simulink model "system2"  (R2023b)
settings: Solver=FixedStepAuto  StartTime=0.0  StopTime=Tmdl  FixedStep=Tmdl/n_steps  RelTol=1e-3
undefined symbols (not defined in the file): x1_initial, x2_initial, x3_initial
settings Model: Creator=deniskirbaba  LastModifiedBy=deniskirbaba

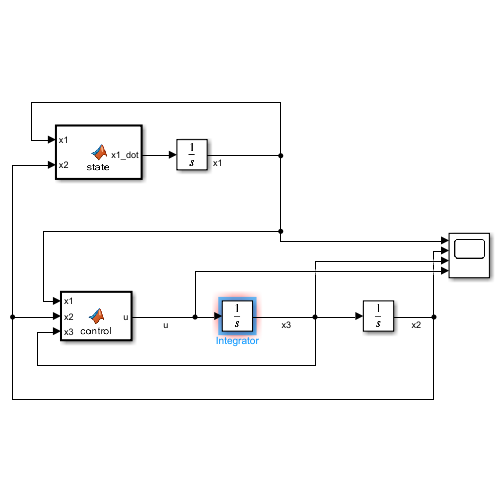
[thumbnail: Simulink's stored preview of the top-level diagram]
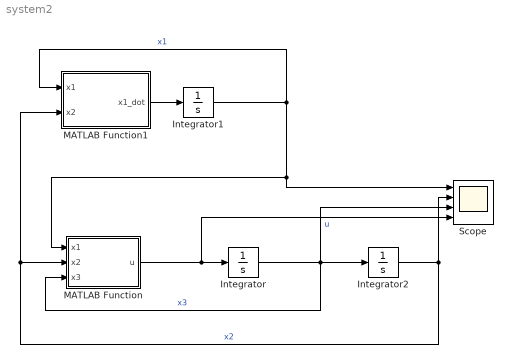
== system system2 ==
  Integrator : Integrator  InitialCondition=x3_initial
  Integrator1 : Integrator  InitialCondition=x1_initial
  Integrator2 : Integrator  InitialCondition=x2_initial
  MATLAB Function : MATLAB Function  TreatAsAtomicUnit=on
  MATLAB Function1 : MATLAB Function  TreatAsAtomicUnit=on
  Scope : Scope  NumInputPorts=4
  wires:
  Integrator/1 -> Integrator2/1, Scope/3, MATLAB Function/3(x3)  "x3"
  MATLAB Function1/1(x1_dot) -> Integrator1/1
  Integrator1/1 -> Scope/1, MATLAB Function/1(x1), MATLAB Function1/1(x1)  "x1"
  MATLAB Function/1(u) -> Scope/4, Integrator/1  "u"
  Integrator2/1 -> MATLAB Function1/2(x2), MATLAB Function/2(x2), Scope/2  "x2"

== matlab function system2/MATLAB Function ==
  data: x1 input; u output; x2 input; x3 input
function u = control(x1,x2,x3)
z2 = x2+1.5*x1^2-x1;
z3 = x3 - (-z2 + (-2*x1+1)*(-x1-0.5*x1^3-z2));
u = -z3 - (x2+1.5*x1^2-x1) + x3*(-1-(1-2*x1)) + (1-3*x1-2*(-x2-1.5*x1^2-0.5*x1^3)+(-2*x1+1)*(-3*x1-1.5*x1^2))*(-x2-1.5*x1^2-0.5*x1^3);

== matlab function system2/MATLAB Function1 ==
  data: x1 input; x1_dot output; x2 input
function x1_dot = state(x1,x2)

x1_dot = -x2-1.5*x1^2-0.5*x1^3;
